simulink model "chap05"  (R2021a)
settings: Solver=FixedStepDiscrete  StartTime=0.0  StopTime=inf  FixedStep=0.001  RelTol=1e-3
undefined symbols (not defined in the file): DiscIntNeverNeededParam, Header, Pose, X, Y, Z
libraries: robotlib x31
(part 4 of 9)

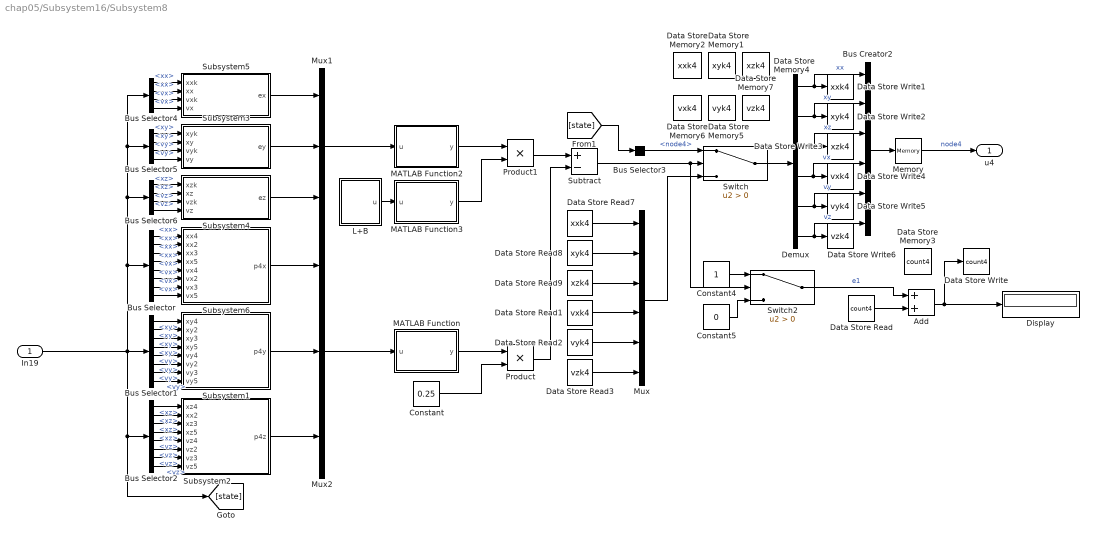
== system chap05/Subsystem16/Subsystem8 ==
  In19 : Inport
  Add : Sum
  Bus Creator2 : BusCreator  Inputs=6
  Bus Selector : BusSelector  OutputSignals=state(tk).node4.xx,state(tk).node2.xx,state(tk).node3.xx,state(tk).node5.xx,state(tk).node4.vx,state(tk).node2.vx,state(tk).node3.vx,state(tk).node5.vx
  Bus Selector1 : BusSelector  OutputSignals=state(tk).node4.xy,state(tk).node2.xy,state(tk).node3.xy,state(tk).node5.xy,state(tk).node4.vy,state(tk).node2.vy,state(tk).node3.vy,state(tk).node5.vy
  Bus Selector2 : BusSelector  OutputSignals=state(tk).node4.xz,state(tk).node2.xz,state(tk).node3.xz,state(tk).node5.xz,state(tk).node4.vz,state(tk).node2.vz,state(tk).node3.vz,state(tk).node5.vz
  Bus Selector3 : BusSelector  OutputSignals=state(t).node4
  Bus Selector4 : BusSelector  OutputSignals=state(tk).node4.xx,state(t).node4.xx,state(tk).node4.vx,state(t).node4.vx
  Bus Selector5 : BusSelector  OutputSignals=state(tk).node4.xy,state(t).node4.xy,state(tk).node4.vy,state(t).node4.vy
  Bus Selector6 : BusSelector  OutputSignals=state(tk).node4.xz,state(t).node4.xz,state(tk).node4.vz,state(t).node4.vz
  Constant : Constant  Value=0.25
  Constant4 : Constant
  Constant5 : Constant  Value=0
  Data Store Memory1 : DataStoreMemory  DataStoreName=xyk4  ReadBeforeWriteMsg=warning  WriteAfterWriteMsg=warning  WriteAfterReadMsg=warning  ShowAdditionalParam=off
  Data Store Memory2 : DataStoreMemory  DataStoreName=xxk4  ReadBeforeWriteMsg=warning  WriteAfterWriteMsg=warning  WriteAfterReadMsg=warning  ShowAdditionalParam=off
  Data Store Memory3 : DataStoreMemory  DataStoreName=count4  ReadBeforeWriteMsg=warning  WriteAfterWriteMsg=warning  WriteAfterReadMsg=warning  ShowAdditionalParam=off
  Data Store Memory4 : DataStoreMemory  DataStoreName=xzk4  ReadBeforeWriteMsg=warning  WriteAfterWriteMsg=warning  WriteAfterReadMsg=warning  ShowAdditionalParam=off
  Data Store Memory5 : DataStoreMemory  DataStoreName=vyk4  ReadBeforeWriteMsg=warning  WriteAfterWriteMsg=warning  WriteAfterReadMsg=warning  ShowAdditionalParam=off
  Data Store Memory6 : DataStoreMemory  DataStoreName=vxk4  ReadBeforeWriteMsg=warning  WriteAfterWriteMsg=warning  WriteAfterReadMsg=warning  ShowAdditionalParam=off
  Data Store Memory7 : DataStoreMemory  DataStoreName=vzk4  ReadBeforeWriteMsg=warning  WriteAfterWriteMsg=warning  WriteAfterReadMsg=warning  ShowAdditionalParam=off
  Data Store Read : DataStoreRead  DataStoreName=count4  IndexOptions=Index vector (dialog)  Indices=1  OutputSizes=1
  Data Store Read1 : DataStoreRead  DataStoreName=vxk4  IndexOptions=Index vector (dialog)  Indices=1  OutputSizes=1
  Data Store Read2 : DataStoreRead  DataStoreName=vyk4  IndexOptions=Index vector (dialog)  Indices=1  OutputSizes=1
  Data Store Read3 : DataStoreRead  DataStoreName=vzk4  IndexOptions=Index vector (dialog)  Indices=1  OutputSizes=1
  Data Store Read7 : DataStoreRead  DataStoreName=xxk4  IndexOptions=Index vector (dialog)  Indices=1  OutputSizes=1
  Data Store Read8 : DataStoreRead  DataStoreName=xyk4  IndexOptions=Index vector (dialog)  Indices=1  OutputSizes=1
  Data Store Read9 : DataStoreRead  DataStoreName=xzk4  IndexOptions=Index vector (dialog)  Indices=1  OutputSizes=1
  Data Store Write : DataStoreWrite  DataStoreName=count4  IndexOptions=Index vector (dialog)  Indices=1  OutputSizes=1
  Data Store Write1 : DataStoreWrite  DataStoreName=xxk4  IndexOptions=Index vector (dialog)  Indices=1  OutputSizes=1
  Data Store Write2 : DataStoreWrite  DataStoreName=xyk4  IndexOptions=Index vector (dialog)  Indices=1  OutputSizes=1
  Data Store Write3 : DataStoreWrite  DataStoreName=xzk4  IndexOptions=Index vector (dialog)  Indices=1  OutputSizes=1
  Data Store Write4 : DataStoreWrite  DataStoreName=vxk4  IndexOptions=Index vector (dialog)  Indices=1  OutputSizes=1
  Data Store Write5 : DataStoreWrite  DataStoreName=vyk4  IndexOptions=Index vector (dialog)  Indices=1  OutputSizes=1
  Data Store Write6 : DataStoreWrite  DataStoreName=vzk4  IndexOptions=Index vector (dialog)  Indices=1  OutputSizes=1
  Demux : Demux  Outputs=6
  Display : Display
  L+B : Subsystem
  MATLAB Function : MATLAB Function  TreatAsAtomicUnit=on
  MATLAB Function2 : MATLAB Function  TreatAsAtomicUnit=on
  MATLAB Function3 : MATLAB Function  TreatAsAtomicUnit=on
  Memory : Memory
  Mux : Mux  Inputs=6
  Mux1 : Mux  Inputs=3
  Mux2 : Mux  Inputs=3
  Product : Product
  Product1 : Product
  Subsystem1 : Subsystem
  Subsystem2 : Subsystem
  Subsystem3 : Subsystem
  Subsystem4 : Subsystem
  Subsystem5 : Subsystem
  Subsystem6 : Subsystem
  Subtract : Sum  Inputs=+-
  Switch : Switch  Criteria=u2 > Threshold
  Switch2 : Switch  Criteria=u2 > Threshold
  u4 : Outport
  wires:
  Subsystem2/1(p4z) -> Mux2/3
  Subsystem6/1(p4x) -> Mux2/1
  Subsystem1/1(p4y) -> Mux2/2
  Bus Selector/1 -> Subsystem6/1(xx4)  "<xx>"
  Bus Selector/2 -> Subsystem6/2(xx2)  "<xx>"
  Bus Selector/3 -> Subsystem6/3(xx3)  "<xx>"
  Bus Selector/4 -> Subsystem6/4(xx5)  "<xx>"
  Bus Selector/5 -> Subsystem6/5(vx4)  "<vx>"
  Bus Selector/6 -> Subsystem6/6(vx2)  "<vx>"
  Bus Selector/7 -> Subsystem6/7(vx3)  "<vx>"
  Bus Selector/8 -> Subsystem6/8(vx5)  "<vx>"
  Bus Selector1/1 -> Subsystem1/1(xy4)  "<xy>"
  Bus Selector1/2 -> Subsystem1/2(xy2)  "<xy>"
  Bus Selector1/3 -> Subsystem1/3(xy3)  "<xy>"
  Bus Selector1/4 -> Subsystem1/4(xy5)  "<xy>"
  Bus Selector1/5 -> Subsystem1/5(vy4)  "<vy>"
  Bus Selector1/6 -> Subsystem1/6(vy2)  "<vy>"
  Bus Selector1/7 -> Subsystem1/7(vy3)  "<vy>"
  Bus Selector1/8 -> Subsystem1/8(vy5)  "<vy>"
  Bus Selector2/1 -> Subsystem2/1(xz4)  "<xz>"
  Bus Selector2/2 -> Subsystem2/2(xx2)  "<xz>"
  Bus Selector2/3 -> Subsystem2/3(xz3)  "<xz>"
  Bus Selector2/4 -> Subsystem2/4(xz5)  "<xz>"
  Bus Selector2/5 -> Subsystem2/5(vz4)  "<vz>"
  Bus Selector2/6 -> Subsystem2/6(vz2)  "<vz>"
  Bus Selector2/7 -> Subsystem2/7(vz3)  "<vz>"
  Bus Selector2/8 -> Subsystem2/8(vz5)  "<vz>"
  Data Store Read3/1 -> Mux/6
  Switch/1 -> Demux/1
  Demux/2 -> Bus Creator2/2, Data Store Write2/1  "xy"
  Bus Selector3/1 -> Switch/1  "<node4>"
  Demux/1 -> Bus Creator2/1, Data Store Write1/1  "xx"
  Switch2/1 -> Add/1  "e1"
  Demux/6 -> Bus Creator2/6, Data Store Write6/1  "vz"
  Demux/3 -> Bus Creator2/3, Data Store Write3/1  "xz"
  Data Store Read7/1 -> Mux/1
  Constant4/1 -> Switch2/1
  Mux/1 -> Switch/3
  Data Store Read9/1 -> Mux/3
  Add/1 -> Data Store Write/1, Display/1
  Demux/4 -> Bus Creator2/4, Data Store Write4/1  "vx"
  Bus Creator2/1 -> Memory/1
  Data Store Read2/1 -> Mux/5
  Data Store Read1/1 -> Mux/4
  Product/1 -> Subtract/2
  Data Store Read8/1 -> Mux/2
  [state] -> Bus Selector3/1
  MATLAB Function3/1(y) -> Product1/2
  Mux1/1 -> MATLAB Function2/1(u)
  Constant5/1 -> Switch2/3
  Constant/1 -> Product/2
  MATLAB Function2/1(y) -> Product1/1
  L+B/1(u) -> MATLAB Function3/1(u)
  Subsystem4/1(ez) -> Mux1/3
  Subsystem5/1(ex) -> Mux1/1
  Subsystem3/1(ey) -> Mux1/2
  Demux/5 -> Bus Creator2/5, Data Store Write5/1  "vy"
  Product1/1 -> Subtract/1
  Data Store Read/1 -> Add/2
  MATLAB Function/1(y) -> Product/1
  Mux2/1 -> MATLAB Function/1(u)
  Bus Selector5/3 -> Subsystem3/3(vyk)  "<vy>"
  In19/1 -> [state], Bus Selector2/1, Bus Selector1/1, Bus Selector/1, Bus Selector6/1, Bus Selector5/1, Bus Selector4/1
  Bus Selector5/2 -> Subsystem3/2(xy)  "<xy>"
  Bus Selector5/4 -> Subsystem3/4(vy)  "<vy>"
  Bus Selector5/1 -> Subsystem3/1(xyk)  "<xy>"
  Bus Selector6/2 -> Subsystem4/2(xz)  "<xz>"
  Bus Selector6/3 -> Subsystem4/3(vzk)  "<vz>"
  Bus Selector6/4 -> Subsystem4/4(vz)  "<vz>"
  Bus Selector6/1 -> Subsystem4/1(xzk)  "<xz>"
  Memory/1 -> u4/1  "node4"
  Bus Selector4/1 -> Subsystem5/1(xxk)  "<xx>"
  Bus Selector4/2 -> Subsystem5/2(xx)  "<xx>"
  Bus Selector4/3 -> Subsystem5/3(vxk)  "<vx>"
  Bus Selector4/4 -> Subsystem5/4(vx)  "<vx>"
  Subtract/1 -> Switch/2, Switch2/2

== system chap05/Gazebo/Subsystem1/Subsystem3 ==
  In1 : Inport
  Constant13 : Constant  Value=-5
  Subtract : Sum
  Out1 : Outport
  wires:
  In1/1 -> Subtract/1
  Subtract/1 -> Out1/1
  Constant13/1 -> Subtract/2

== system chap05/Gazebo/Subsystem2/Subsystem3 ==
  In1 : Inport
  Constant13 : Constant  Value=-6
  Subtract : Sum
  Out1 : Outport
  wires:
  In1/1 -> Subtract/1
  Subtract/1 -> Out1/1
  Constant13/1 -> Subtract/2

== system chap05/Gazebo/Subsystem2/Subsystem4 ==
  In1 : Inport
  Constant13 : Constant
  Subtract : Sum
  Out1 : Outport
  wires:
  Constant13/1 -> Subtract/2
  Subtract/1 -> Out1/1
  In1/1 -> Subtract/1

== system chap05/Gazebo/Subsystem3/Subsystem3 ==
  In1 : Inport
  Constant13 : Constant  Value=-5
  Subtract : Sum
  Out1 : Outport
  wires:
  In1/1 -> Subtract/1
  Subtract/1 -> Out1/1
  Constant13/1 -> Subtract/2

== system chap05/Gazebo/Subsystem3/Subsystem4 ==
  In1 : Inport
  Constant13 : Constant
  Subtract : Sum
  Out1 : Outport
  wires:
  Constant13/1 -> Subtract/2
  Subtract/1 -> Out1/1
  In1/1 -> Subtract/1

== system chap05/Gazebo/Subsystem4/Subsystem1 ==
  In1 : Inport
  Constant13 : Constant  Value=-4
  Subtract : Sum
  Out1 : Outport
  wires:
  In1/1 -> Subtract/1
  Subtract/1 -> Out1/1
  Constant13/1 -> Subtract/2

== system chap05/Gazebo/Subsystem4/Subsystem2 ==
  In1 : Inport
  Constant13 : Constant
  Subtract : Sum
  Out1 : Outport
  wires:
  Constant13/1 -> Subtract/2
  Subtract/1 -> Out1/1
  In1/1 -> Subtract/1

== system chap05/Gazebo/Subsystem5/Subsystem1 ==
  In1 : Inport
  Constant13 : Constant  Value=-6
  Subtract : Sum
  Out1 : Outport
  wires:
  In1/1 -> Subtract/1
  Subtract/1 -> Out1/1
  Constant13/1 -> Subtract/2

== system chap05/Gazebo/Subsystem5/Subsystem2 ==
  In1 : Inport
  Constant13 : Constant  Value=-1
  Subtract : Sum
  Out1 : Outport
  wires:
  Constant13/1 -> Subtract/2
  Subtract/1 -> Out1/1
  In1/1 -> Subtract/1

== system chap05/Gazebo/Subsystem6/Subsystem1 ==
  In1 : Inport
  Constant13 : Constant  Value=-5
  Subtract : Sum
  Out1 : Outport
  wires:
  In1/1 -> Subtract/1
  Subtract/1 -> Out1/1
  Constant13/1 -> Subtract/2

== system chap05/Gazebo/Subsystem6/Subsystem2 ==
  In1 : Inport
  Constant13 : Constant  Value=-1
  Subtract : Sum
  Out1 : Outport
  wires:
  Constant13/1 -> Subtract/2
  Subtract/1 -> Out1/1
  In1/1 -> Subtract/1

== system chap05/Gazebo/Subsystem7/Subsystem1 ==
  In1 : Inport
  Constant13 : Constant  Value=-4
  Subtract : Sum
  Out1 : Outport
  wires:
  In1/1 -> Subtract/1
  Subtract/1 -> Out1/1
  Constant13/1 -> Subtract/2

== system chap05/Gazebo/Subsystem7/Subsystem2 ==
  In1 : Inport
  Constant13 : Constant  Value=-1
  Subtract : Sum
  Out1 : Outport
  wires:
  Constant13/1 -> Subtract/2
  Subtract/1 -> Out1/1
  In1/1 -> Subtract/1

== system chap05/Subsystem16/Subsystem/Subsystem1 ==
  xy1 : Inport
  xy2 : Inport  Port=2
  xy3 : Inport  Port=3
  xy6 : Inport  Port=4
  vy1 : Inport  Port=5
  vy2 : Inport  Port=6
  vy3 : Inport  Port=7
  vy6 : Inport  Port=8
  Add : Sum
  Add{1,4,6,8} (4 alike) : Sum  Inputs=-+
  Add2 : Sum  Inputs=+-
  Add5 : Sum  Inputs=+++
  Add7 : Sum  Inputs=+-
  Add9 : Sum  Inputs=+++
  Constant : Constant  Value=0.75
  Constant1 : Constant  Value=0.85
  Constant3 : Constant  Value=0.5
  Constant4 : Constant  Value=0.8
  Constant5 : Constant  Value=1.2
  Constant7 : Constant  Value=0.5
  Constant8 : Constant  Value=0.8
  Constant9 : Constant  Value=1.2
  Gain : Gain  Gain=-1
  Product{1,3..9} (8 alike) : Product
  utx : Outport
  wires:
  Product8/1 -> Add9/2
  Product9/1 -> Add9/3
  Constant7/1 -> Product8/1
  Add8/1 -> Product8/2
  vy1/1 -> Add6/2, Add8/2, Add7/1
  Constant8/1 -> Product9/2
  Add7/1 -> Product9/1
  vy3/1 -> Add8/1
  vy2/1 -> Add7/2
  vy6/1 -> Add6/1
  Constant9/1 -> Product7/1
  Add6/1 -> Product7/2
  Product7/1 -> Add9/1
  Product3/1 -> Add5/1
  Add1/1 -> Product3/2
  Constant5/1 -> Product3/1
  xy6/1 -> Add1/1
  xy2/1 -> Add2/2
  xy3/1 -> Add4/1
  Add5/1 -> Product6/2
  Add2/1 -> Product5/1
  Product1/1 -> Add/2
  Constant1/1 -> Product1/1
  Constant/1 -> Product6/1
  Product6/1 -> Add/1
  Constant4/1 -> Product5/2
  xy1/1 -> Add2/1, Add4/2, Add1/2
  Add4/1 -> Product4/2
  Constant3/1 -> Product4/1
  Product5/1 -> Add5/3
  Product4/1 -> Add5/2
  Add9/1 -> Product1/2
  Gain/1 -> utx/1
  Add/1 -> Gain/1

== system chap05/Subsystem16/Subsystem/Subsystem10 ==
  utx : Inport
  uty : Inport  Port=2
  utz : Inport  Port=3
  Add : Sum
  Constant3 : Constant
  Constant4 : Constant  Value=0
  Data Store Memory : DataStoreMemory  DataStoreName=utkz1  ReadBeforeWriteMsg=warning  WriteAfterWriteMsg=warning  WriteAfterReadMsg=warning  ShowAdditionalParam=off
  Data Store Memory1 : DataStoreMemory  DataStoreName=utky1  ReadBeforeWriteMsg=warning  WriteAfterWriteMsg=warning  WriteAfterReadMsg=warning  ShowAdditionalParam=off
  Data Store Memory2 : DataStoreMemory  DataStoreName=utkx1  ReadBeforeWriteMsg=warning  WriteAfterWriteMsg=warning  WriteAfterReadMsg=warning  ShowAdditionalParam=off
  Data Store Memory3 : DataStoreMemory  DataStoreName=uc1  ReadBeforeWriteMsg=warning  WriteAfterWriteMsg=warning  WriteAfterReadMsg=warning  ShowAdditionalParam=off
  Data Store Read : DataStoreRead  DataStoreName=uc1  IndexOptions=Index vector (dialog)  Indices=1  OutputSizes=1
  Data Store Read4 : DataStoreRead  DataStoreName=utkx1  IndexOptions=Index vector (dialog)  Indices=1  OutputSizes=1
  Data Store Read5 : DataStoreRead  DataStoreName=utky1  IndexOptions=Index vector (dialog)  Indices=1  OutputSizes=1
  Data Store Read6 : DataStoreRead  DataStoreName=utkz1  IndexOptions=Index vector (dialog)  Indices=1  OutputSizes=1
  Data Store Write : DataStoreWrite  DataStoreName=uc1  IndexOptions=Index vector (dialog)  Indices=1  OutputSizes=1
  Data Store Write1 : DataStoreWrite  DataStoreName=utkx1  IndexOptions=Index vector (dialog)  Indices=1  OutputSizes=1
  Data Store Write2 : DataStoreWrite  DataStoreName=utky1  IndexOptions=Index vector (dialog)  Indices=1  OutputSizes=1
  Data Store Write6 : DataStoreWrite  DataStoreName=utkz1  IndexOptions=Index vector (dialog)  Indices=1  OutputSizes=1
  Demux : Demux  Outputs=3
  Display : Display
  MATLAB Function : MATLAB Function  TreatAsAtomicUnit=on
  Mux1 : Mux  Inputs=3
  Mux2 : Mux  Inputs=3
  Switch : Switch  Threshold=0.1
  Switch2 : Switch  Threshold=0.1
  ux : Outport
  uy : Outport  Port=2
  uz : Outport  Port=3
  wires:
  Switch/1 -> Demux/1
  Data Store Read4/1 -> Mux2/1
  Data Store Read6/1 -> Mux2/3
  Data Store Read5/1 -> Mux2/2
  Demux/3 -> Data Store Write6/1, uz/1
  Demux/1 -> Data Store Write1/1, ux/1
  Add/1 -> Data Store Write/1, Display/1
  Data Store Read/1 -> Add/2
  Switch2/1 -> Add/1  "e1"
  Constant3/1 -> Switch2/1
  Constant4/1 -> Switch2/3
  utx/1 -> Mux1/1
  uty/1 -> Mux1/2
  utz/1 -> Mux1/3
  Demux/2 -> Data Store Write2/1, uy/1
  [ut] -> Switch/1
  [utk] -> Switch/3
  MATLAB Function/1(nrom) -> Switch2/2, Switch/2
  Mux1/1 -> [ut], MATLAB Function/1(u)
  Mux2/1 -> [utk], MATLAB Function/2(utk)

== system chap05/Subsystem16/Subsystem/Subsystem11 ==
  vz1 : Inport
  utz : Inport  Port=2
  gain : Inport  Port=3
  switch : Inport  Port=4
  Add1 : Sum  Inputs=--+
  Constant1 : Constant  Value=0.08
  Constant2 : Constant  Value=10
  Product : Product
  Product1 : Product
  Product2 : Product
  Subsystem : Subsystem
  Subtract : Sum  Inputs=+-
  Switch1 : Switch  Criteria=u2 > Threshold  Threshold=1
  Tanh : Trigonometry  Operator=tanh
  uz : Outport
  Sz : Outport  Port=2
  wires:
  utz/1 -> [A], Subsystem/2(zt3)
  Product/1 -> Add1/2
  vz1/1 -> Subtract/1
  Product2/1 -> Tanh/1
  Tanh/1 -> Product/1
  gain/1 -> Product/2
  [A] -> Add1/3
  Constant2/1 -> Product2/2
  Product1/1 -> Add1/1
  Constant1/1 -> Product1/1
  Subtract/1 -> Sz/1, Product1/2, Product2/1
  Subsystem/1(Out1) -> Subtract/2
  switch/1 -> [switch], Subsystem/1(switch)
  Switch1/1 -> uz/1
  Add1/1 -> Switch1/1
  [A] -> Switch1/3
  [switch] -> Switch1/2

== system chap05/Subsystem16/Subsystem/Subsystem2 ==
  xz1 : Inport
  xx2 : Inport  Port=2
  xz3 : Inport  Port=3
  xz6 : Inport  Port=4
  vz1 : Inport  Port=5
  vz2 : Inport  Port=6
  vz3 : Inport  Port=7
  vz6 : Inport  Port=8
  Add : Sum
  Add{1,4,6,8} (4 alike) : Sum  Inputs=-+
  Add2 : Sum  Inputs=+-
  Add5 : Sum  Inputs=+++
  Add7 : Sum  Inputs=+-
  Add9 : Sum  Inputs=+++
  Constant : Constant  Value=0.75
  Constant1 : Constant  Value=0.85
  Constant3 : Constant  Value=0.5
  Constant4 : Constant  Value=0.8
  Constant5 : Constant  Value=1.2
  Constant7 : Constant  Value=0.5
  Constant8 : Constant  Value=0.8
  Constant9 : Constant  Value=1.2
  Gain : Gain  Gain=-1
  Product{1,3..9} (8 alike) : Product
  utx : Outport
  wires:
  Add9/1 -> Product1/2
  Product4/1 -> Add5/2
  Product5/1 -> Add5/3
  Constant3/1 -> Product4/1
  Add4/1 -> Product4/2
  xz1/1 -> Add1/2, Add4/2, Add2/1
  Constant4/1 -> Product5/2
  Product6/1 -> Add/1
  Constant/1 -> Product6/1
  Constant1/1 -> Product1/1
  Product1/1 -> Add/2
  Add2/1 -> Product5/1
  Add5/1 -> Product6/2
  xz3/1 -> Add4/1
  xx2/1 -> Add2/2
  xz6/1 -> Add1/1
  Constant5/1 -> Product3/1
  Add1/1 -> Product3/2
  Product3/1 -> Add5/1
  Product7/1 -> Add9/1
  Add6/1 -> Product7/2
  Constant9/1 -> Product7/1
  vz6/1 -> Add6/1
  vz2/1 -> Add7/2
  vz3/1 -> Add8/1
  Add7/1 -> Product9/1
  Constant8/1 -> Product9/2
  vz1/1 -> Add7/1, Add8/2, Add6/2
  Add8/1 -> Product8/2
  Constant7/1 -> Product8/1
  Product9/1 -> Add9/3
  Product8/1 -> Add9/2
  Gain/1 -> utx/1
  Add/1 -> Gain/1

== system chap05/Subsystem16/Subsystem/Subsystem3 ==
  utx : Inport
  vx : Inport  Port=2
  vy : Inport  Port=3
  vz : Inport  Port=4
  uty : Inport  Port=5
  ux : Inport  Port=6
  uy : Inport  Port=7
  uz : Inport  Port=8
  utz : Inport  Port=9
  switch : Inport  Port=10
  Add3 : Sum  Inputs=-+
  Add4 : Sum  Inputs=-+
  Add5 : Sum  Inputs=-+
  Demux : Demux  Outputs=3
  Demux1 : Demux  Outputs=3
  Discrete-Time Integrator1 : DiscreteIntegrator  SampleTime=-1  ICPrevOutput=DiscIntNeverNeededParam  ICPrevScaledInput=DiscIntNeverNeededParam
  Discrete-Time Integrator2 : DiscreteIntegrator  SampleTime=-1  ICPrevOutput=DiscIntNeverNeededParam  ICPrevScaledInput=DiscIntNeverNeededParam
  Discrete-Time Integrator8 : DiscreteIntegrator  SampleTime=-1  ICPrevOutput=DiscIntNeverNeededParam  ICPrevScaledInput=DiscIntNeverNeededParam
  MATLAB Function : MATLAB Function  TreatAsAtomicUnit=on
  MATLAB Function1 : MATLAB Function  TreatAsAtomicUnit=on
  MATLAB Function2 : MATLAB Function  TreatAsAtomicUnit=on
  Mux : Mux  Inputs=3
  Mux1 : Mux  Inputs=3
  Subsystem : Subsystem
  Subsystem1 : Subsystem
  Subsystem2 : Subsystem
      settings: PortSchema="{\"entries\":[{\"content\":{\"sides\":[{\"content\":{\"connectorIds\":[\"In1\"]},\"type\":\"ConnectorPlacement.EquallySpacedRectSide\",\"uuid\":\"fc08b57d-5108-4bb3-894e-d1527c9ee9b9\"},{\"content\":{\"connectorIds\":[\"Out1\",\"Out2\",\"Out3\",\"Out4\"],\"side\":\"RIGHT\"},\"type\":\"ConnectorPlacement.EquallySpacedRectSide\",\"uuid\":\"5f28f464-9d6d-4ee7-848e-113b4b51ead6\"},{\"content\":{\"connectorIds\":[],\"side\":\"TOP\"},\"type\":\"ConnectorPlacement.EquallySpacedRectSide\",\"uuid\":\"5cca314e-822b-43eb-ac4d-78622e8ed582\"},{\"content\":{\"connectorIds\":[\"In2\"],\"side\":\"BOTTOM\"},\"type\":\"ConnectorPlacement.EquallySpacedRectSide\",\"uuid\":\"aa07b2d0-4f6e-4d8e-96de-14c35ee3da88\"}]},\"type\":\"ConnectorPlacement.EquallySpacedConnector\",\"uuid\":\"246d6f2c-2f9e-403c-b810-eff9b0fc0735\"}],\"packageUris\":[\"http://schema.mathworks.com/mf0/Connector/R2020b\"],\"version\":\"1.0\"}"
  Subsystem3 : Subsystem
  Subtract1 : Sum  Inputs=++++
  Subtract2 : Sum  Inputs=+-
  Subtract3 : Sum  Inputs=+-
  Subtract4 : Sum  Inputs=+-
  Switch1 : Switch  Criteria=u2 > Threshold  Threshold=1
  Switch2 : Switch  Criteria=u2 > Threshold  Threshold=1
  Switch3 : Switch  Criteria=u2 > Threshold  Threshold=1
  udtx : Outport
  udty : Outport  Port=2
  udtz : Outport  Port=3
  wires:
  Subsystem3/1(Out1) -> Subtract1/2
  Subsystem2/2(k2) -> Subsystem3/2(k2)
  Subsystem1/1(Out1) -> Subtract1/1
  Subsystem2/1(k1) -> Subsystem1/2(k1)
  Subtract4/1 -> MATLAB Function2/1(u)
  Subtract3/1 -> MATLAB Function1/1(u)
  Subtract2/1 -> MATLAB Function/1(u)
  Demux/3 -> Discrete-Time Integrator8/1
  Demux/1 -> Discrete-Time Integrator2/1
  Demux/2 -> Discrete-Time Integrator1/1
  Discrete-Time Integrator2/1 -> Subtract2/1
  Discrete-Time Integrator1/1 -> Subtract3/1
  Discrete-Time Integrator8/1 -> Subtract4/1
  Mux1/1 -> Subtract1/4
  ux/1 -> Mux1/1
  uy/1 -> Mux1/2
  uz/1 -> Mux1/3
  vx/1 -> Subtract2/2
  Subsystem2/4(k4) -> Subsystem/3(k4)
  Subsystem/1(z2) -> Subtract1/3, Demux1/1  "od1"
  Subsystem2/3(k3) -> Subsystem/2(k3)
  Subtract1/1 -> Demux/1
  Mux/1 -> Subsystem1/1(e1), Subsystem3/1(e1), Subsystem2/1(e1), Subsystem/1(e1)
  utx/1 -> Switch1/3, Add3/2
  uty/1 -> Switch2/3, Add5/2
  utz/1 -> Switch3/3, Add4/2
  vy/1 -> Subtract3/2
  vz/1 -> Subtract4/2
  MATLAB Function/1(y) -> Mux/1
  MATLAB Function1/1(y) -> Mux/2
  MATLAB Function2/1(y) -> Mux/3
  switch/1 -> [switch], Switch3/2, Switch2/2, Switch1/2
  [switch] -> Subsystem2/2(switch)
  Add3/1 -> Switch1/1
  Add5/1 -> Switch2/1
  Add4/1 -> Switch3/1
  Switch1/1 -> udtx/1
  Switch2/1 -> udty/1
  Switch3/1 -> udtz/1
  Demux1/3 -> Add4/1
  Demux1/2 -> Add5/1
  Demux1/1 -> Add3/1

== system chap05/Subsystem16/Subsystem/Subsystem4 ==
  vx1 : Inport
  utx : Inport  Port=2
  gain : Inport  Port=3
  switch : Inport  Port=4
  Add1 : Sum  Inputs=--+
  Constant1 : Constant  Value=0.08
  Constant2 : Constant  Value=10
  Product : Product
  Product1 : Product
  Product2 : Product
  Subsystem : Subsystem
  Subtract : Sum  Inputs=+-
  Switch1 : Switch  Criteria=u2 > Threshold  Threshold=1
  Tanh : Trigonometry  Operator=tanh
  ux : Outport
  Sx : Outport  Port=2
  wires:
  Add1/1 -> Switch1/1
  utx/1 -> [A], Subsystem/2(zt3)
  Product/1 -> Add1/2
  vx1/1 -> Subtract/1
  Product2/1 -> Tanh/1
  Tanh/1 -> Product/1
  gain/1 -> Product/2
  [A] -> Add1/3
  Constant2/1 -> Product2/2
  Product1/1 -> Add1/1
  Constant1/1 -> Product1/1
  Subtract/1 -> Sx/1, Product1/2, Product2/1
  switch/1 -> [switch], Subsystem/1(switch)
  [A] -> Switch1/3
  [switch] -> Switch1/2
  Switch1/1 -> ux/1
  Subsystem/1(Out1) -> Subtract/2

== system chap05/Subsystem16/Subsystem/Subsystem6 ==
  xx1 : Inport
  xx2 : Inport  Port=2
  xx3 : Inport  Port=3
  xx6 : Inport  Port=4
  vx1 : Inport  Port=5
  vx2 : Inport  Port=6
  vx3 : Inport  Port=7
  vx6 : Inport  Port=8
  Add : Sum
  Add{1,4,6,8} (4 alike) : Sum  Inputs=-+
  Add2 : Sum  Inputs=+-
  Add5 : Sum  Inputs=+++
  Add7 : Sum  Inputs=+-
  Add9 : Sum  Inputs=+++
  Constant : Constant  Value=0.75
  Constant1 : Constant  Value=0.85
  Constant3 : Constant  Value=0.5
  Constant4 : Constant  Value=0.8
  Constant5 : Constant  Value=1.2
  Constant7 : Constant  Value=0.5
  Constant8 : Constant  Value=0.8
  Constant9 : Constant  Value=1.2
  Gain : Gain  Gain=-1
  Product{1,3..9} (8 alike) : Product
  utx : Outport
  wires:
  Add9/1 -> Product1/2
  Product4/1 -> Add5/2
  Product5/1 -> Add5/3
  Constant3/1 -> Product4/1
  Add4/1 -> Product4/2
  xx1/1 -> Add1/2, Add4/2, Add2/1
  Constant4/1 -> Product5/2
  Product6/1 -> Add/1
  Constant/1 -> Product6/1
  Constant1/1 -> Product1/1
  Product1/1 -> Add/2
  Add2/1 -> Product5/1
  Add5/1 -> Product6/2
  xx3/1 -> Add4/1
  xx2/1 -> Add2/2
  xx6/1 -> Add1/1
  Constant5/1 -> Product3/1
  Add1/1 -> Product3/2
  Product3/1 -> Add5/1
  Product7/1 -> Add9/1
  Add6/1 -> Product7/2
  Constant9/1 -> Product7/1
  vx6/1 -> Add6/1
  vx2/1 -> Add7/2
  vx3/1 -> Add8/1
  Add7/1 -> Product9/1
  Constant8/1 -> Product9/2
  vx1/1 -> Add7/1, Add8/2, Add6/2
  Add8/1 -> Product8/2
  Constant7/1 -> Product8/1
  Product9/1 -> Add9/3
  Product8/1 -> Add9/2
  Add/1 -> Gain/1
  Gain/1 -> utx/1

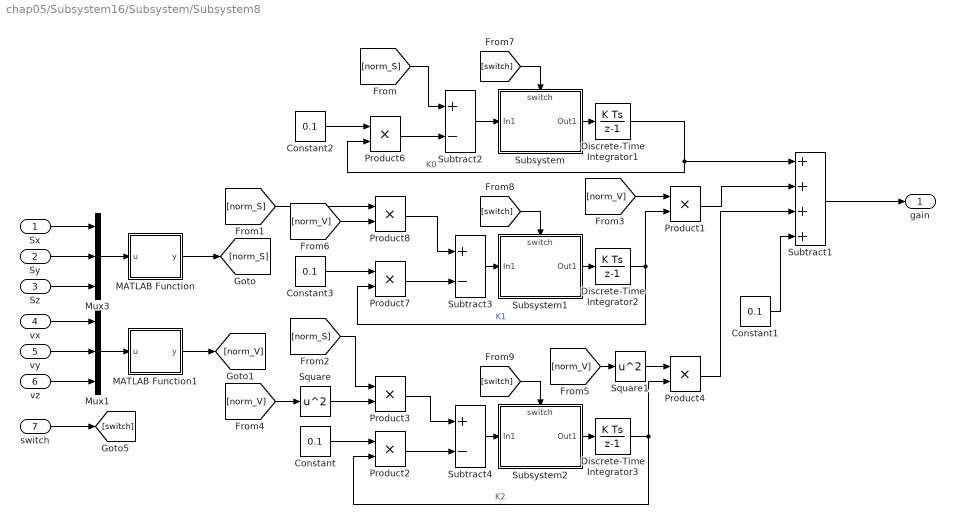
== system chap05/Subsystem16/Subsystem/Subsystem8 ==
  Sx : Inport
  Sy : Inport  Port=2
  Sz : Inport  Port=3
  vx : Inport  Port=4
  vy : Inport  Port=5
  vz : Inport  Port=6
  switch : Inport  Port=7
  Constant{,1..3} (4 alike) : Constant  Value=0.1
  Discrete-Time Integrator1 : DiscreteIntegrator  gainval=1  InitialCondition=0.05  SampleTime=-1  ICPrevOutput=DiscIntNeverNeededParam  ICPrevScaledInput=DiscIntNeverNeededParam
  Discrete-Time Integrator2 : DiscreteIntegrator  gainval=1  InitialCondition=0.025  SampleTime=-1  ICPrevOutput=DiscIntNeverNeededParam  ICPrevScaledInput=DiscIntNeverNeededParam
  Discrete-Time Integrator3 : DiscreteIntegrator  gainval=1  InitialCondition=0.01  SampleTime=-1  ICPrevOutput=DiscIntNeverNeededParam  ICPrevScaledInput=DiscIntNeverNeededParam
  MATLAB Function : MATLAB Function  TreatAsAtomicUnit=on
  MATLAB Function1 : MATLAB Function  TreatAsAtomicUnit=on
  Mux1 : Mux  Inputs=3
  Mux3 : Mux  Inputs=3
  Product{1..4,6..8} (7 alike) : Product
  Square : Math  Operator=square  SaturateOnIntegerOverflow=on
  Square1 : Math  Operator=square  SaturateOnIntegerOverflow=on
  Subsystem : Subsystem
      settings: PortSchema="{\"entries\":[{\"content\":{\"sides\":[{\"content\":{\"connectorIds\":[\"In1\"]},\"type\":\"ConnectorPlacement.EquallySpacedRectSide\",\"uuid\":\"50b1559e-7173-4ba8-93e6-314f6d9df527\"},{\"content\":{\"connectorIds\":[\"Out1\"],\"side\":\"RIGHT\"},\"type\":\"ConnectorPlacement.EquallySpacedRectSide\",\"uuid\":\"be527bac-0bcc-4faf-a185-0382edae0189\"},{\"content\":{\"connectorIds\":[\"In2\"],\"side\":\"TOP\"},\"type\":\"ConnectorPlacement.EquallySpacedRectSide\",\"uuid\":\"4c8ef68d-7cf5-4d15-9758-89dbc1169805\"}]},\"type\":\"ConnectorPlacement.EquallySpacedConnector\",\"uuid\":\"3c2ee67b-c3c9-431a-8107-6d5cd22b236e\"}],\"packageUris\":[\"http://schema.mathworks.com/mf0/Connector/R2020b\"],\"version\":\"1.0\"}"
  Subsystem1 : Subsystem
      settings: PortSchema="{\"entries\":[{\"content\":{\"sides\":[{\"content\":{\"connectorIds\":[\"In1\"]},\"type\":\"ConnectorPlacement.EquallySpacedRectSide\",\"uuid\":\"50b1559e-7173-4ba8-93e6-314f6d9df527\"},{\"content\":{\"connectorIds\":[\"Out1\"],\"side\":\"RIGHT\"},\"type\":\"ConnectorPlacement.EquallySpacedRectSide\",\"uuid\":\"be527bac-0bcc-4faf-a185-0382edae0189\"},{\"content\":{\"connectorIds\":[\"In2\"],\"side\":\"TOP\"},\"type\":\"ConnectorPlacement.EquallySpacedRectSide\",\"uuid\":\"4c8ef68d-7cf5-4d15-9758-89dbc1169805\"}]},\"type\":\"ConnectorPlacement.EquallySpacedConnector\",\"uuid\":\"3c2ee67b-c3c9-431a-8107-6d5cd22b236e\"}],\"packageUris\":[\"http://schema.mathworks.com/mf0/Connector/R2020b\"],\"version\":\"1.0\"}"
  Subsystem2 : Subsystem
      settings: PortSchema="{\"entries\":[{\"content\":{\"sides\":[{\"content\":{\"connectorIds\":[\"In1\"]},\"type\":\"ConnectorPlacement.EquallySpacedRectSide\",\"uuid\":\"50b1559e-7173-4ba8-93e6-314f6d9df527\"},{\"content\":{\"connectorIds\":[\"Out1\"],\"side\":\"RIGHT\"},\"type\":\"ConnectorPlacement.EquallySpacedRectSide\",\"uuid\":\"be527bac-0bcc-4faf-a185-0382edae0189\"},{\"content\":{\"connectorIds\":[\"In2\"],\"side\":\"TOP\"},\"type\":\"ConnectorPlacement.EquallySpacedRectSide\",\"uuid\":\"4c8ef68d-7cf5-4d15-9758-89dbc1169805\"}]},\"type\":\"ConnectorPlacement.EquallySpacedConnector\",\"uuid\":\"3c2ee67b-c3c9-431a-8107-6d5cd22b236e\"}],\"packageUris\":[\"http://schema.mathworks.com/mf0/Connector/R2020b\"],\"version\":\"1.0\"}"
  Subtract1 : Sum  Inputs=++++
  Subtract2 : Sum  Inputs=+-
  Subtract3 : Sum  Inputs=+-
  Subtract4 : Sum  Inputs=+-
  " gain" : Outport
  wires:
  [switch] -> Subsystem2/2(switch)
  [switch] -> Subsystem1/2(switch)
  [switch] -> Subsystem/2(switch)
  switch/1 -> [switch]
  Subsystem1/1(Out1) -> Discrete-Time Integrator2/1
  Subsystem2/1(Out1) -> Discrete-Time Integrator3/1
  Subsystem/1(Out1) -> Discrete-Time Integrator1/1
  [norm_V] -> Product8/2
  Square1/1 -> Product4/1
  [norm_V] -> Square1/1
  [norm_V] -> Product1/1
  [norm_V] -> Square/1
  [norm_S] -> Product3/1
  [norm_S] -> Product8/1
  [norm_S] -> Subtract2/1
  MATLAB Function/1(y) -> [norm_S]
  vy/1 -> Mux1/2
  vz/1 -> Mux1/3
  vx/1 -> Mux1/1
  Sz/1 -> Mux3/3
  Sy/1 -> Mux3/2
  Sx/1 -> Mux3/1
  Constant3/1 -> Product7/1
  Constant2/1 -> Product6/1
  Constant1/1 -> Subtract1/4
  Product4/1 -> Subtract1/3
  MATLAB Function1/1(y) -> [norm_V]
  Constant/1 -> Product2/1
  Mux1/1 -> MATLAB Function1/1(u)
  Square/1 -> Product3/2
  Mux3/1 -> MATLAB Function/1(u)
  Discrete-Time Integrator3/1 -> Product2/2, Product4/2  "K2"
  Product2/1 -> Subtract4/2
  Product3/1 -> Subtract4/1
  Subtract4/1 -> Subsystem2/1(In1)
  Subtract3/1 -> Subsystem1/1(In1)
  Product8/1 -> Subtract3/1
  Product7/1 -> Subtract3/2
  Discrete-Time Integrator2/1 -> Product1/2, Product7/2  "K1"
  Product6/1 -> Subtract2/2
  Discrete-Time Integrator1/1 -> Subtract1/1, Product6/2  "K0"
  Subtract2/1 -> Subsystem/1(In1)
  Product1/1 -> Subtract1/2
  Subtract1/1 -> " gain"/1

== system chap05/Subsystem16/Subsystem/Subsystem9 ==
  vy1 : Inport
  uty : Inport  Port=2
  gain : Inport  Port=3
  switch : Inport  Port=4
  Add1 : Sum  Inputs=--+
  Constant1 : Constant  Value=0.08
  Constant2 : Constant  Value=10
  Product : Product
  Product1 : Product
  Product2 : Product
  Subsystem : Subsystem
  Subtract : Sum  Inputs=+-
  Switch1 : Switch  Criteria=u2 > Threshold  Threshold=1
  Tanh : Trigonometry  Operator=tanh
  uy : Outport
  Sz : Outport  Port=2
  wires:
  Switch1/1 -> uy/1
  switch/1 -> Subsystem/1(switch), [switch]
  Subtract/1 -> Product2/1, Product1/2, Sz/1
  Constant1/1 -> Product1/1
  Product1/1 -> Add1/1
  Constant2/1 -> Product2/2
  [A] -> Add1/3
  gain/1 -> Product/2
  Tanh/1 -> Product/1
  Product2/1 -> Tanh/1
  vy1/1 -> Subtract/1
  Product/1 -> Add1/2
  uty/1 -> Subsystem/2(zt3), [A]
  Subsystem/1(Out1) -> Subtract/2
  Add1/1 -> Switch1/1
  [A] -> Switch1/3
  [switch] -> Switch1/2

== system chap05/Subsystem16/Subsystem1/Subsystem1 ==
  xy5 : Inport
  xy0 : Inport  Port=2
  xy3 : Inport  Port=3
  xy4 : Inport  Port=4
  vy5 : Inport  Port=5
  vy0 : Inport  Port=6
  vy3 : Inport  Port=7
  vy4 : Inport  Port=8
  Add : Sum
  Add1 : Sum  Inputs=-+
  Add10 : Sum  Inputs=-+
  Add2 : Sum  Inputs=+-
  Add4 : Sum  Inputs=-+
  Add5 : Sum  Inputs=+++
  Add6 : Sum  Inputs=+-
  Add8 : Sum  Inputs=+++
  Add9 : Sum  Inputs=+-
  Constant : Constant  Value=0.75
  Constant1 : Constant  Value=0.85
  Constant3 : Constant  Value=1.2
  Constant{4,6..8} (4 alike) : Constant  Value=1.5
  Constant5 : Constant  Value=1.2
  Gain : Gain  Gain=-1
  Product{1,3..9} (8 alike) : Product
  uty : Outport
  wires:
  vy0/1 -> Add6/2
  Constant8/1 -> Product7/2
  Add6/1 -> Product7/1
  Product7/1 -> Add8/3
  Product3/1 -> Add5/1
  xy0/1 -> Add1/1
  Add1/1 -> Product3/2
  Constant7/1 -> Product3/1
  Product9/1 -> Add8/2
  Product8/1 -> Add8/1
  Add9/1 -> Product9/1
  Constant6/1 -> Product9/2
  Add10/1 -> Product8/2
  Constant5/1 -> Product8/1
  Add8/1 -> Product1/2
  Product4/1 -> Add5/2
  Product5/1 -> Add5/3
  Constant3/1 -> Product4/1
  Add4/1 -> Product4/2
  xy5/1 -> Add2/1, Add4/2, Add1/2
  Constant4/1 -> Product5/2
  Product6/1 -> Add/1
  Constant/1 -> Product6/1
  Constant1/1 -> Product1/1
  Product1/1 -> Add/2
  Add2/1 -> Product5/1
  Add5/1 -> Product6/2
  xy4/1 -> Add4/1
  xy3/1 -> Add2/2
  vy3/1 -> Add9/2
  vy4/1 -> Add10/1
  vy5/1 -> Add9/1, Add6/1, Add10/2
  Gain/1 -> uty/1
  Add/1 -> Gain/1

== system chap05/Subsystem16/Subsystem1/Subsystem10 ==
  utx : Inport
  uty : Inport  Port=2
  utz : Inport  Port=3
  Add : Sum
  Constant3 : Constant
  Constant4 : Constant  Value=0
  Data Store Memory : DataStoreMemory  DataStoreName=utkz5  ReadBeforeWriteMsg=warning  WriteAfterWriteMsg=warning  WriteAfterReadMsg=warning  ShowAdditionalParam=off
  Data Store Memory1 : DataStoreMemory  DataStoreName=utky5  ReadBeforeWriteMsg=warning  WriteAfterWriteMsg=warning  WriteAfterReadMsg=warning  ShowAdditionalParam=off
  Data Store Memory2 : DataStoreMemory  DataStoreName=utkx5  ReadBeforeWriteMsg=warning  WriteAfterWriteMsg=warning  WriteAfterReadMsg=warning  ShowAdditionalParam=off
  Data Store Memory3 : DataStoreMemory  DataStoreName=uc5  ReadBeforeWriteMsg=warning  WriteAfterWriteMsg=warning  WriteAfterReadMsg=warning  ShowAdditionalParam=off
  Data Store Read : DataStoreRead  DataStoreName=uc5  IndexOptions=Index vector (dialog)  Indices=1  OutputSizes=1
  Data Store Read1 : DataStoreRead  DataStoreName=utkz5  IndexOptions=Index vector (dialog)  Indices=1  OutputSizes=1
  Data Store Read2 : DataStoreRead  DataStoreName=utky5  IndexOptions=Index vector (dialog)  Indices=1  OutputSizes=1
  Data Store Read3 : DataStoreRead  DataStoreName=utkx5  IndexOptions=Index vector (dialog)  Indices=1  OutputSizes=1
  Data Store Write : DataStoreWrite  DataStoreName=uc5  IndexOptions=Index vector (dialog)  Indices=1  OutputSizes=1
  Data Store Write3 : DataStoreWrite  DataStoreName=utkx5  IndexOptions=Index vector (dialog)  Indices=1  OutputSizes=1
  Data Store Write4 : DataStoreWrite  DataStoreName=utky5  IndexOptions=Index vector (dialog)  Indices=1  OutputSizes=1
  Data Store Write5 : DataStoreWrite  DataStoreName=utkz5  IndexOptions=Index vector (dialog)  Indices=1  OutputSizes=1
  Demux : Demux  Outputs=3
  Display : Display
  MATLAB Function : MATLAB Function  TreatAsAtomicUnit=on
  Mux1 : Mux  Inputs=3
  Mux2 : Mux  Inputs=3
  Switch : Switch  Threshold=0.1
  Switch2 : Switch  Threshold=0.1
  ux : Outport
  uy : Outport  Port=2
  uz : Outport  Port=3
  wires:
  Mux2/1 -> [utk], MATLAB Function/2(utk)
  Mux1/1 -> [ut], MATLAB Function/1(u)
  Switch/1 -> Demux/1
  Data Store Read3/1 -> Mux2/1
  Data Store Read1/1 -> Mux2/3
  Data Store Read2/1 -> Mux2/2
  Demux/3 -> Data Store Write5/1, uz/1
  Demux/1 -> Data Store Write3/1, ux/1
  Add/1 -> Data Store Write/1, Display/1
  Data Store Read/1 -> Add/2
  Switch2/1 -> Add/1  "e1"
  Constant3/1 -> Switch2/1
  Constant4/1 -> Switch2/3
  MATLAB Function/1(nrom) -> Switch2/2, Switch/2
  utx/1 -> Mux1/1
  uty/1 -> Mux1/2
  utz/1 -> Mux1/3
  Demux/2 -> Data Store Write4/1, uy/1
  [ut] -> Switch/1
  [utk] -> Switch/3

== system chap05/Subsystem16/Subsystem1/Subsystem11 ==
  vz5 : Inport
  vz0 : Inport  Port=2
  utz : Inport  Port=3
  gain : Inport  Port=4
  switch : Inport  Port=5
  Add1 : Sum  Inputs=--+
  Constant1 : Constant  Value=0.08
  Constant2 : Constant  Value=10
  Product : Product
  Product1 : Product
  Product2 : Product
  Subsystem : Subsystem
  Subtract : Sum  Inputs=+--
  Switch1 : Switch  Criteria=u2 > Threshold  Threshold=1
  Tanh : Trigonometry  Operator=tanh
  uz : Outport
  Sz : Outport  Port=2
  wires:
  Add1/1 -> Switch1/1
  utz/1 -> [A], Subsystem/2(zt3)
  Subsystem/1(Out1) -> Subtract/3
  Product/1 -> Add1/2
  vz5/1 -> Subtract/1
  Product2/1 -> Tanh/1
  Tanh/1 -> Product/1
  gain/1 -> Product/2
  [A] -> Add1/3
  Constant2/1 -> Product2/2
  Product1/1 -> Add1/1
  Subtract/1 -> Sz/1, Product1/2, Product2/1
  vz0/1 -> Subtract/2
  switch/1 -> [switch], Subsystem/1(switch)
  [A] -> Switch1/3
  [switch] -> Switch1/2
  Switch1/1 -> uz/1
  Constant1/1 -> Product1/1

== system chap05/Subsystem16/Subsystem1/Subsystem2 ==
  xz5 : Inport
  xz0 : Inport  Port=2
  xz3 : Inport  Port=3
  xz4 : Inport  Port=4
  vz5 : Inport  Port=5
  vz0 : Inport  Port=6
  vz3 : Inport  Port=7
  vz4 : Inport  Port=8
  Add : Sum
  Add1 : Sum  Inputs=-+
  Add10 : Sum  Inputs=-+
  Add2 : Sum  Inputs=+-
  Add4 : Sum  Inputs=-+
  Add5 : Sum  Inputs=+++
  Add6 : Sum  Inputs=+-
  Add8 : Sum  Inputs=+++
  Add9 : Sum  Inputs=+-
  Constant : Constant  Value=0.75
  Constant1 : Constant  Value=0.85
  Constant3 : Constant  Value=1.2
  Constant{4,6..8} (4 alike) : Constant  Value=1.5
  Constant5 : Constant  Value=1.2
  Gain : Gain  Gain=-1
  Product{1,3..9} (8 alike) : Product
  utz : Outport
  wires:
  vz5/1 -> Add10/2, Add6/1, Add9/1
  vz4/1 -> Add10/1
  vz3/1 -> Add9/2
  xz3/1 -> Add2/2
  xz4/1 -> Add4/1
  Add5/1 -> Product6/2
  Add2/1 -> Product5/1
  Product1/1 -> Add/2
  Constant1/1 -> Product1/1
  Constant/1 -> Product6/1
  Product6/1 -> Add/1
  Constant4/1 -> Product5/2
  xz5/1 -> Add1/2, Add4/2, Add2/1
  Add4/1 -> Product4/2
  Constant3/1 -> Product4/1
  Product5/1 -> Add5/3
  Product4/1 -> Add5/2
  Add8/1 -> Product1/2
  Constant5/1 -> Product8/1
  Add10/1 -> Product8/2
  Constant6/1 -> Product9/2
  Add9/1 -> Product9/1
  Product8/1 -> Add8/1
  Product9/1 -> Add8/2
  Constant7/1 -> Product3/1
  Add1/1 -> Product3/2
  xz0/1 -> Add1/1
  Product3/1 -> Add5/1
  Product7/1 -> Add8/3
  Add6/1 -> Product7/1
  Constant8/1 -> Product7/2
  vz0/1 -> Add6/2
  Gain/1 -> utz/1
  Add/1 -> Gain/1

== system chap05/Subsystem16/Subsystem1/Subsystem3 ==
  utx : Inport
  vx : Inport  Port=2
  vy : Inport  Port=3
  vz : Inport  Port=4
  uty : Inport  Port=5
  ux : Inport  Port=6
  uy : Inport  Port=7
  uz : Inport  Port=8
  utz : Inport  Port=9
  switch : Inport  Port=10
  Add3 : Sum  Inputs=-+
  Add4 : Sum  Inputs=-+
  Add5 : Sum  Inputs=-+
  Demux : Demux  Outputs=3
  Demux1 : Demux  Outputs=3
  Discrete-Time Integrator1 : DiscreteIntegrator  SampleTime=-1  ICPrevOutput=DiscIntNeverNeededParam  ICPrevScaledInput=DiscIntNeverNeededParam
  Discrete-Time Integrator2 : DiscreteIntegrator  SampleTime=-1  ICPrevOutput=DiscIntNeverNeededParam  ICPrevScaledInput=DiscIntNeverNeededParam
  Discrete-Time Integrator8 : DiscreteIntegrator  SampleTime=-1  ICPrevOutput=DiscIntNeverNeededParam  ICPrevScaledInput=DiscIntNeverNeededParam
  MATLAB Function : MATLAB Function  TreatAsAtomicUnit=on
  MATLAB Function1 : MATLAB Function  TreatAsAtomicUnit=on
  MATLAB Function2 : MATLAB Function  TreatAsAtomicUnit=on
  Mux : Mux  Inputs=3
  Mux1 : Mux  Inputs=3
  Subsystem : Subsystem
  Subsystem1 : Subsystem
  Subsystem2 : Subsystem
      settings: PortSchema="{\"entries\":[{\"content\":{\"sides\":[{\"content\":{\"connectorIds\":[\"In1\"]},\"type\":\"ConnectorPlacement.EquallySpacedRectSide\",\"uuid\":\"fc08b57d-5108-4bb3-894e-d1527c9ee9b9\"},{\"content\":{\"connectorIds\":[\"Out1\",\"Out2\",\"Out3\",\"Out4\"],\"side\":\"RIGHT\"},\"type\":\"ConnectorPlacement.EquallySpacedRectSide\",\"uuid\":\"5f28f464-9d6d-4ee7-848e-113b4b51ead6\"},{\"content\":{\"connectorIds\":[],\"side\":\"TOP\"},\"type\":\"ConnectorPlacement.EquallySpacedRectSide\",\"uuid\":\"5cca314e-822b-43eb-ac4d-78622e8ed582\"},{\"content\":{\"connectorIds\":[\"In2\"],\"side\":\"BOTTOM\"},\"type\":\"ConnectorPlacement.EquallySpacedRectSide\",\"uuid\":\"aa07b2d0-4f6e-4d8e-96de-14c35ee3da88\"}]},\"type\":\"ConnectorPlacement.EquallySpacedConnector\",\"uuid\":\"246d6f2c-2f9e-403c-b810-eff9b0fc0735\"}],\"packageUris\":[\"http://schema.mathworks.com/mf0/Connector/R2020b\"],\"version\":\"1.0\"}"
  Subsystem3 : Subsystem
  Subtract1 : Sum  Inputs=++++
  Subtract2 : Sum  Inputs=+-
  Subtract3 : Sum  Inputs=+-
  Subtract4 : Sum  Inputs=+-
  Switch1 : Switch  Criteria=u2 > Threshold  Threshold=1
  Switch2 : Switch  Criteria=u2 > Threshold  Threshold=1
  Switch3 : Switch  Criteria=u2 > Threshold  Threshold=1
  udtx : Outport
  udty : Outport  Port=2
  udtz : Outport  Port=3
  wires:
  Subsystem3/1(Out1) -> Subtract1/2
  Subsystem2/2(k2) -> Subsystem3/2(k2)
  Subsystem1/1(Out1) -> Subtract1/1
  Subsystem2/1(k1) -> Subsystem1/2(k1)
  Subtract4/1 -> MATLAB Function2/1(u)
  Subtract3/1 -> MATLAB Function1/1(u)
  Subtract2/1 -> MATLAB Function/1(u)
  Demux/3 -> Discrete-Time Integrator8/1
  Demux/1 -> Discrete-Time Integrator2/1
  Demux/2 -> Discrete-Time Integrator1/1
  Discrete-Time Integrator2/1 -> Subtract2/1
  Discrete-Time Integrator1/1 -> Subtract3/1
  Discrete-Time Integrator8/1 -> Subtract4/1
  Mux1/1 -> Subtract1/4
  ux/1 -> Mux1/1
  uy/1 -> Mux1/2
  uz/1 -> Mux1/3
  vx/1 -> Subtract2/2
  Subsystem2/4(k4) -> Subsystem/3(k4)
  Subsystem/1(z2) -> Subtract1/3, Demux1/1  "od5"
  Subsystem2/3(k3) -> Subsystem/2(k3)
  Subtract1/1 -> Demux/1
  Mux/1 -> Subsystem1/1(e1), Subsystem3/1(e1), Subsystem2/1(e1), Subsystem/1(e1)
  utx/1 -> Switch1/3, Add3/2
  uty/1 -> Switch2/3, Add5/2
  utz/1 -> Switch3/3, Add4/2
  vy/1 -> Subtract3/2
  vz/1 -> Subtract4/2
  MATLAB Function/1(y) -> Mux/1
  MATLAB Function1/1(y) -> Mux/2
  MATLAB Function2/1(y) -> Mux/3
  switch/1 -> [switch], Switch3/2, Switch1/2, Switch2/2
  [switch] -> Subsystem2/2(switch)
  Add3/1 -> Switch1/1
  Add5/1 -> Switch2/1
  Add4/1 -> Switch3/1
  Switch1/1 -> udtx/1
  Switch2/1 -> udty/1
  Switch3/1 -> udtz/1
  Demux1/1 -> Add3/1
  Demux1/2 -> Add5/1
  Demux1/3 -> Add4/1

== system chap05/Subsystem16/Subsystem1/Subsystem5 ==
  vx5 : Inport
  vx0 : Inport  Port=2
  utx : Inport  Port=3
  gain : Inport  Port=4
  switch : Inport  Port=5
  Add1 : Sum  Inputs=--+
  Constant1 : Constant  Value=0.08
  Constant2 : Constant  Value=10
  Product : Product
  Product1 : Product
  Product2 : Product
  Subsystem : Subsystem
  Subtract : Sum  Inputs=+--
  Switch1 : Switch  Criteria=u2 > Threshold  Threshold=1
  Tanh : Trigonometry  Operator=tanh
  ux : Outport
  Sx : Outport  Port=2
  wires:
  Add1/1 -> Switch1/1
  utx/1 -> [A], Subsystem/2(zt3)
  Subsystem/1(Out1) -> Subtract/3
  Product/1 -> Add1/2
  vx5/1 -> Subtract/1
  Product2/1 -> Tanh/1
  Tanh/1 -> Product/1
  gain/1 -> Product/2
  [A] -> Add1/3
  Constant2/1 -> Product2/2
  Product1/1 -> Add1/1
  Subtract/1 -> Sx/1, Product1/2, Product2/1
  vx0/1 -> Subtract/2
  switch/1 -> [switch], Subsystem/1(switch)
  [A] -> Switch1/3
  [switch] -> Switch1/2
  Switch1/1 -> ux/1
  Constant1/1 -> Product1/1

== system chap05/Subsystem16/Subsystem1/Subsystem6 ==
  xx5 : Inport
  xx0 : Inport  Port=2
  xx3 : Inport  Port=3
  xx4 : Inport  Port=4
  vx5 : Inport  Port=5
  vx0 : Inport  Port=6
  vx3 : Inport  Port=7
  vx4 : Inport  Port=8
  Add : Sum
  Add1 : Sum  Inputs=-+
  Add10 : Sum  Inputs=-+
  Add2 : Sum  Inputs=+-
  Add4 : Sum  Inputs=-+
  Add5 : Sum  Inputs=+++
  Add6 : Sum  Inputs=+-
  Add8 : Sum  Inputs=+++
  Add9 : Sum  Inputs=+-
  Constant : Constant  Value=0.75
  Constant1 : Constant  Value=0.85
  Constant3 : Constant  Value=1.2
  Constant{4,6..8} (4 alike) : Constant  Value=1.5
  Constant5 : Constant  Value=1.2
  Gain : Gain  Gain=-1
  Product{1,3..9} (8 alike) : Product
  utx : Outport
  wires:
  vx5/1 -> Add10/2, Add6/1, Add9/1
  vx4/1 -> Add10/1
  vx3/1 -> Add9/2
  xx3/1 -> Add2/2
  xx4/1 -> Add4/1
  Add5/1 -> Product6/2
  Add2/1 -> Product5/1
  Product1/1 -> Add/2
  Constant1/1 -> Product1/1
  Constant/1 -> Product6/1
  Product6/1 -> Add/1
  Constant4/1 -> Product5/2
  xx5/1 -> Add1/2, Add4/2, Add2/1
  Add4/1 -> Product4/2
  Constant3/1 -> Product4/1
  Product5/1 -> Add5/3
  Product4/1 -> Add5/2
  Add8/1 -> Product1/2
  Constant5/1 -> Product8/1
  Add10/1 -> Product8/2
  Constant6/1 -> Product9/2
  Add9/1 -> Product9/1
  Product8/1 -> Add8/1
  Product9/1 -> Add8/2
  Constant7/1 -> Product3/1
  Add1/1 -> Product3/2
  xx0/1 -> Add1/1
  Product3/1 -> Add5/1
  Product7/1 -> Add8/3
  Add6/1 -> Product7/1
  Constant8/1 -> Product7/2
  vx0/1 -> Add6/2
  Gain/1 -> utx/1
  Add/1 -> Gain/1

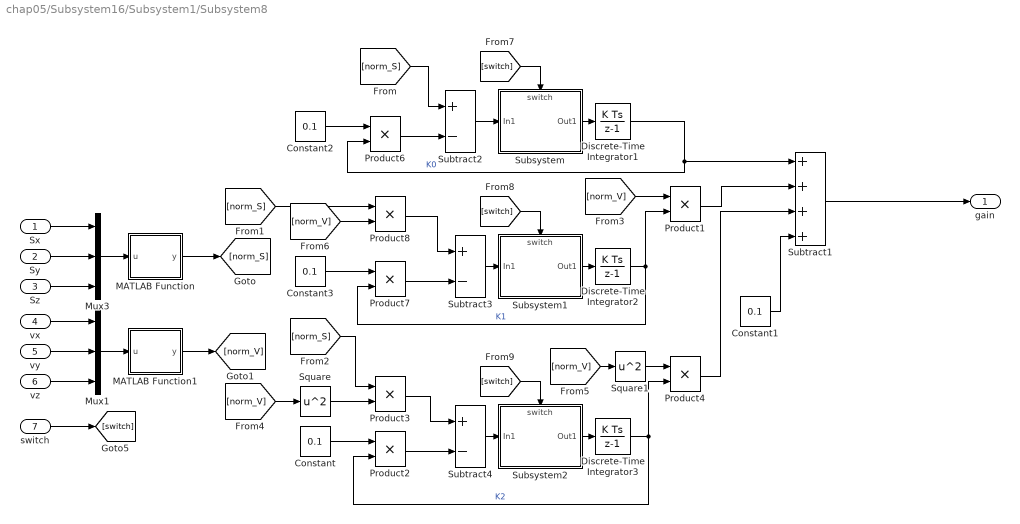
== system chap05/Subsystem16/Subsystem1/Subsystem8 ==
  Sx : Inport
  Sy : Inport  Port=2
  Sz : Inport  Port=3
  vx : Inport  Port=4
  vy : Inport  Port=5
  vz : Inport  Port=6
  switch : Inport  Port=7
  Constant{,1..3} (4 alike) : Constant  Value=0.1
  Discrete-Time Integrator1 : DiscreteIntegrator  gainval=1  InitialCondition=0.05  SampleTime=-1  ICPrevOutput=DiscIntNeverNeededParam  ICPrevScaledInput=DiscIntNeverNeededParam
  Discrete-Time Integrator2 : DiscreteIntegrator  gainval=1  InitialCondition=0.025  SampleTime=-1  ICPrevOutput=DiscIntNeverNeededParam  ICPrevScaledInput=DiscIntNeverNeededParam
  Discrete-Time Integrator3 : DiscreteIntegrator  gainval=1  InitialCondition=0.01  SampleTime=-1  ICPrevOutput=DiscIntNeverNeededParam  ICPrevScaledInput=DiscIntNeverNeededParam
  MATLAB Function : MATLAB Function  TreatAsAtomicUnit=on
  MATLAB Function1 : MATLAB Function  TreatAsAtomicUnit=on
  Mux1 : Mux  Inputs=3
  Mux3 : Mux  Inputs=3
  Product{1..4,6..8} (7 alike) : Product
  Square : Math  Operator=square  SaturateOnIntegerOverflow=on
  Square1 : Math  Operator=square  SaturateOnIntegerOverflow=on
  Subsystem : Subsystem
      settings: PortSchema="{\"entries\":[{\"content\":{\"sides\":[{\"content\":{\"connectorIds\":[\"In1\"]},\"type\":\"ConnectorPlacement.EquallySpacedRectSide\",\"uuid\":\"50b1559e-7173-4ba8-93e6-314f6d9df527\"},{\"content\":{\"connectorIds\":[\"Out1\"],\"side\":\"RIGHT\"},\"type\":\"ConnectorPlacement.EquallySpacedRectSide\",\"uuid\":\"be527bac-0bcc-4faf-a185-0382edae0189\"},{\"content\":{\"connectorIds\":[\"In2\"],\"side\":\"TOP\"},\"type\":\"ConnectorPlacement.EquallySpacedRectSide\",\"uuid\":\"4c8ef68d-7cf5-4d15-9758-89dbc1169805\"}]},\"type\":\"ConnectorPlacement.EquallySpacedConnector\",\"uuid\":\"3c2ee67b-c3c9-431a-8107-6d5cd22b236e\"}],\"packageUris\":[\"http://schema.mathworks.com/mf0/Connector/R2020b\"],\"version\":\"1.0\"}"
  Subsystem1 : Subsystem
      settings: PortSchema="{\"entries\":[{\"content\":{\"sides\":[{\"content\":{\"connectorIds\":[\"In1\"]},\"type\":\"ConnectorPlacement.EquallySpacedRectSide\",\"uuid\":\"50b1559e-7173-4ba8-93e6-314f6d9df527\"},{\"content\":{\"connectorIds\":[\"Out1\"],\"side\":\"RIGHT\"},\"type\":\"ConnectorPlacement.EquallySpacedRectSide\",\"uuid\":\"be527bac-0bcc-4faf-a185-0382edae0189\"},{\"content\":{\"connectorIds\":[\"In2\"],\"side\":\"TOP\"},\"type\":\"ConnectorPlacement.EquallySpacedRectSide\",\"uuid\":\"4c8ef68d-7cf5-4d15-9758-89dbc1169805\"}]},\"type\":\"ConnectorPlacement.EquallySpacedConnector\",\"uuid\":\"3c2ee67b-c3c9-431a-8107-6d5cd22b236e\"}],\"packageUris\":[\"http://schema.mathworks.com/mf0/Connector/R2020b\"],\"version\":\"1.0\"}"
  Subsystem2 : Subsystem
      settings: PortSchema="{\"entries\":[{\"content\":{\"sides\":[{\"content\":{\"connectorIds\":[\"In1\"]},\"type\":\"ConnectorPlacement.EquallySpacedRectSide\",\"uuid\":\"50b1559e-7173-4ba8-93e6-314f6d9df527\"},{\"content\":{\"connectorIds\":[\"Out1\"],\"side\":\"RIGHT\"},\"type\":\"ConnectorPlacement.EquallySpacedRectSide\",\"uuid\":\"be527bac-0bcc-4faf-a185-0382edae0189\"},{\"content\":{\"connectorIds\":[\"In2\"],\"side\":\"TOP\"},\"type\":\"ConnectorPlacement.EquallySpacedRectSide\",\"uuid\":\"4c8ef68d-7cf5-4d15-9758-89dbc1169805\"}]},\"type\":\"ConnectorPlacement.EquallySpacedConnector\",\"uuid\":\"3c2ee67b-c3c9-431a-8107-6d5cd22b236e\"}],\"packageUris\":[\"http://schema.mathworks.com/mf0/Connector/R2020b\"],\"version\":\"1.0\"}"
  Subtract1 : Sum  Inputs=++++
  Subtract2 : Sum  Inputs=+-
  Subtract3 : Sum  Inputs=+-
  Subtract4 : Sum  Inputs=+-
  " gain" : Outport
  wires:
  [switch] -> Subsystem2/2(switch)
  [switch] -> Subsystem1/2(switch)
  [switch] -> Subsystem/2(switch)
  switch/1 -> [switch]
  Subsystem1/1(Out1) -> Discrete-Time Integrator2/1
  Subsystem2/1(Out1) -> Discrete-Time Integrator3/1
  Subsystem/1(Out1) -> Discrete-Time Integrator1/1
  [norm_V] -> Product8/2
  Square1/1 -> Product4/1
  [norm_V] -> Square1/1
  [norm_V] -> Product1/1
  [norm_V] -> Square/1
  [norm_S] -> Product3/1
  [norm_S] -> Product8/1
  [norm_S] -> Subtract2/1
  MATLAB Function/1(y) -> [norm_S]
  vy/1 -> Mux1/2
  vz/1 -> Mux1/3
  vx/1 -> Mux1/1
  Sz/1 -> Mux3/3
  Sy/1 -> Mux3/2
  Sx/1 -> Mux3/1
  Constant3/1 -> Product7/1
  Constant2/1 -> Product6/1
  Constant1/1 -> Subtract1/4
  Product4/1 -> Subtract1/3
  MATLAB Function1/1(y) -> [norm_V]
  Constant/1 -> Product2/1
  Mux1/1 -> MATLAB Function1/1(u)
  Square/1 -> Product3/2
  Mux3/1 -> MATLAB Function/1(u)
  Discrete-Time Integrator3/1 -> Product2/2, Product4/2  "K2"
  Product2/1 -> Subtract4/2
  Product3/1 -> Subtract4/1
  Subtract4/1 -> Subsystem2/1(In1)
  Subtract3/1 -> Subsystem1/1(In1)
  Product8/1 -> Subtract3/1
  Product7/1 -> Subtract3/2
  Discrete-Time Integrator2/1 -> Product1/2, Product7/2  "K1"
  Product6/1 -> Subtract2/2
  Discrete-Time Integrator1/1 -> Subtract1/1, Product6/2  "K0"
  Subtract2/1 -> Subsystem/1(In1)
  Product1/1 -> Subtract1/2
  Subtract1/1 -> " gain"/1

== system chap05/Subsystem16/Subsystem1/Subsystem9 ==
  vy5 : Inport
  vy0 : Inport  Port=2
  uty : Inport  Port=3
  gain : Inport  Port=4
  switch : Inport  Port=5
  Add1 : Sum  Inputs=--+
  Constant1 : Constant  Value=0.08
  Constant2 : Constant  Value=10
  Product : Product
  Product1 : Product
  Product2 : Product
  Subsystem : Subsystem
  Subtract : Sum  Inputs=+--
  Switch1 : Switch  Criteria=u2 > Threshold  Threshold=1
  Tanh : Trigonometry  Operator=tanh
  uy : Outport
  Sz : Outport  Port=2
  wires:
  Switch1/1 -> uy/1
  [switch] -> Switch1/2
  [A] -> Switch1/3
  switch/1 -> Subsystem/1(switch), [switch]
  vy0/1 -> Subtract/2
  Subtract/1 -> Product2/1, Product1/2, Sz/1
  Product1/1 -> Add1/1
  Constant2/1 -> Product2/2
  [A] -> Add1/3
  gain/1 -> Product/2
  Tanh/1 -> Product/1
  Product2/1 -> Tanh/1
  vy5/1 -> Subtract/1
  Product/1 -> Add1/2
  Subsystem/1(Out1) -> Subtract/3
  uty/1 -> Subsystem/2(zt3), [A]
  Add1/1 -> Switch1/1
  Constant1/1 -> Product1/1

== system chap05/Subsystem16/Subsystem12/L+B ==
  Add : Sum
  Constant1 : Constant  Value=|
      | [2.5 0 0 0 0 0
      |      0 2.8 0 0 0 0
      |      0 0 2.8 0 0 0
      |      0 0 0 2.5 0 0
      |      0 0 0 0 2.7 0
      |      0 0 0 0 0 2.7]
  Constant2 : Constant  Value=|
      | [0.0 0.8 0.5 0.0 0.0 1.2
      |      0.8 0.0 0.0 0.5 0.0 1.5
      |      0.5 0.0 0.0 0.8 1.5 0.0
      |      0.0 0.5 0.8 0.0 1.2 0.0
      |      0.0 0.0 1.5 1.2 0.0 0.0
      |      1.2 1.5 0.0 0.0 0.0 0.0]
  Constant3 : Constant  Value=|
      | [0.0 0.0 0.0 0.0 0.0 0.0
      |      0.0 0.0 0.0 0.0 0.0 0.0
      |      0.0 0.0 0.0 0.0 0.0 0.0
      |      0.0 0.0 0.0 0.0 0.0 0.0
      |      0.0 0.0 0.0 0.0 1.5 0.0
      |      0.0 0.0 0.0 0.0 0.0 1.5]
  Subtract : Sum  Inputs=+-
  u : Outport
  wires:
  Constant2/1 -> Subtract/2
  Constant1/1 -> Subtract/1
  Subtract/1 -> Add/1
  Add/1 -> u/1
  Constant3/1 -> Add/2
